simulink model "pathPlanningSimulinkModel"  (R2022b)
settings: Solver=VariableStepAuto  StartTime=0.0  StopTime=inf  RelTol=1e-3
model workspace (MAT data in the model file):
  Sig = Simulink.Signal
  Sig.DataType = 'auto'
  Sig.Dimensions = -1
  Sig.DimensionsMode = 'auto'
  Sig.Complexity = 'auto'
  Sig.SampleTime = -1
  Sig.SamplingMode = 'auto'
values from neighbouring files (symbols this model uses):
  complexMap = [1 1 1 1 1 1 1 1 1 1 1 1 ... (2132 elements, 41x52)]    [matlab.mat]
  r = rateControl(1/sampleTime)    [lidarsensor.m]
undefined symbols (not defined in the file or in its folder): a, b, c, m, n, o, p, q
libraries: robotmobilelib x3, robotalgslib x3
settings Model: Creator=The MathWorks, Inc.  LastModifiedBy=christian.badolo
settings SolverCC: AlgebraicLoopSolver=TrustRegion
settings DebuggingCC: UnconnectedInputMsg=warning  UnconnectedOutputMsg=warning  UnconnectedLineMsg=warning  SymbolicDimsDataTypeCodeGenerationDiagnostic=none  SFMachineParentedDataDiag=warning
settings ModelReferenceCC: EnableRefExpFcnMdlSchedulingChecks=on
settings RTWCC: DLArmComputeVersion=19.05

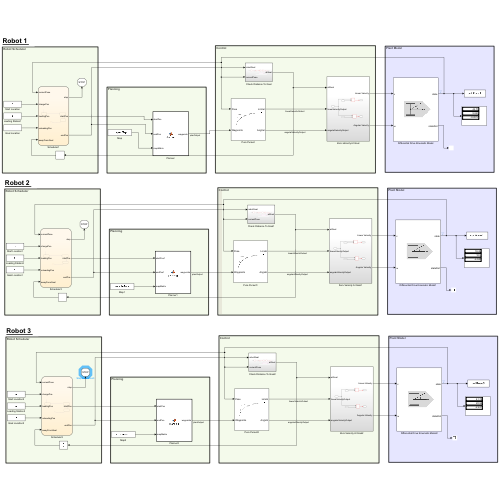
[thumbnail: Simulink's stored preview of the top-level diagram]
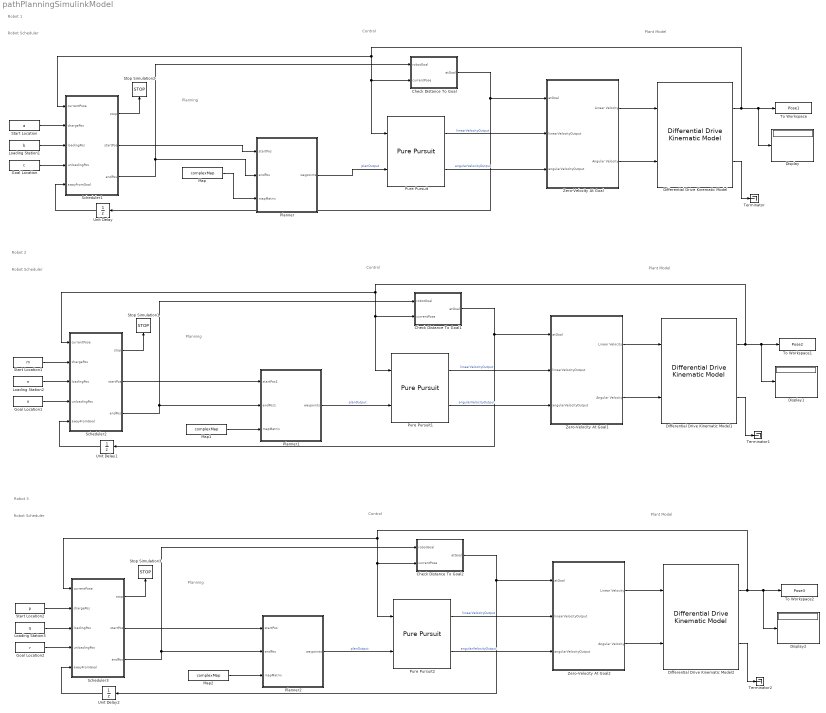
== system pathPlanningSimulinkModel ==
  note: Robot 1
  note: Plant Model
  note: Control
  note: Robot Scheduler
  note: Planning
  note: Plant Model
  note: Planning
  note: Control
  note: Robot Scheduler
  note: Robot 2
  note: Planning
  note: Control
  note: Robot Scheduler
  note: Plant Model
  note: Robot 3
  Check Distance To Goal : Subsystem
  Check Distance To Goal1 : Subsystem
  Check Distance To Goal2 : Subsystem
  Differential Drive Kinematic Model : robotmobilelib/Differential Drive Kinematic Model  VehicleInputs=Vehicle Speed & Heading Angular Velocity  WheelRadius=0.05  WheelSpeedRange=[-inf inf]  TrackWidth=0.2  InitialState=[a, 0]'  SimulateUsing=Interpreted execution
  Differential Drive Kinematic Model1 : robotmobilelib/Differential Drive Kinematic Model  VehicleInputs=Vehicle Speed & Heading Angular Velocity  WheelRadius=0.05  WheelSpeedRange=[-inf inf]  TrackWidth=0.2  InitialState=[m, 0]'  SimulateUsing=Interpreted execution
  Differential Drive Kinematic Model2 : robotmobilelib/Differential Drive Kinematic Model  VehicleInputs=Vehicle Speed & Heading Angular Velocity  WheelRadius=0.05  WheelSpeedRange=[-inf inf]  TrackWidth=0.2  InitialState=[p, 0]'  SimulateUsing=Interpreted execution
  Display : Display
  Display1 : Display
  Display2 : Display
  Goal Location : Constant  Value=c
  Goal Location1 : Constant  Value=o
  Goal Location2 : Constant  Value=r
  Loading Station1 : Constant  Value=b
  Loading Station2 : Constant  Value=n
  Loading Station3 : Constant  Value=q
  Map : Constant  Value=complexMap
  Map1 : Constant  Value=complexMap
  Map2 : Constant  Value=complexMap
  Planner : MATLAB Function  TreatAsAtomicUnit=on
  Planner1 : MATLAB Function  TreatAsAtomicUnit=on
  Planner2 : MATLAB Function  TreatAsAtomicUnit=on
  Pure Pursuit : robotalgslib/Pure Pursuit  DesiredLinearVelocity=0.5  MaxAngularVelocity=1.0  LookaheadDistance=0.5  TargetDirPort=off  SimulateUsing=Code generation
  Pure Pursuit1 : robotalgslib/Pure Pursuit  DesiredLinearVelocity=0.5  MaxAngularVelocity=1.0  LookaheadDistance=0.5  TargetDirPort=off  SimulateUsing=Code generation
  Pure Pursuit2 : robotalgslib/Pure Pursuit  DesiredLinearVelocity=0.2  MaxAngularVelocity=1.0  LookaheadDistance=0.5  TargetDirPort=off  SimulateUsing=Code generation
  Scheduler1 : Stateflow chart  TreatAsAtomicUnit=on
  Scheduler2 : Stateflow chart  TreatAsAtomicUnit=on
  Scheduler3 : Stateflow chart  TreatAsAtomicUnit=on
  Start Location : Constant  Value=a
  Start Location1 : Constant  Value=m
  Start Location2 : Constant  Value=p
  Stop Simulation1 : Stop
  Stop Simulation2 : Stop
  Stop Simulation3 : Stop
  Terminator : Terminator
  Terminator1 : Terminator
  Terminator2 : Terminator
  To Workspace : ToWorkspace  VariableName=Pose1  SampleTime=-1
  To Workspace1 : ToWorkspace  VariableName=Pose2  SampleTime=-1
  To Workspace2 : ToWorkspace  VariableName=Pose3  SampleTime=-1
  Unit Delay : UnitDelay  SampleTime=-1  HasFrameUpgradeWarning=on
  Unit Delay1 : UnitDelay  SampleTime=-1  HasFrameUpgradeWarning=on
  Unit Delay2 : UnitDelay  SampleTime=-1  HasFrameUpgradeWarning=on
  Zero-Velocity At Goal : Subsystem
  Zero-Velocity At Goal1 : Subsystem
  Zero-Velocity At Goal2 : Subsystem
  wires:
  Check Distance To Goal/1(atGoal) -> Unit Delay/1, Zero-Velocity At Goal/1(atGoal)
  Pure Pursuit/1 -> Zero-Velocity At Goal/2(linearVelocityOutput)  "linearVelocityOutput"
  Planner/1(waypoints) -> Pure Pursuit/2  "planOutput"
  Pure Pursuit/2 -> Zero-Velocity At Goal/3(angularVelocityOutput)  "angularVelocityOutput"
  Zero-Velocity At Goal/1(Linear Velocity) -> Differential Drive Kinematic Model/1
  Zero-Velocity At Goal/2(Angular Velocity) -> Differential Drive Kinematic Model/2
  Differential Drive Kinematic Model/2 -> Terminator/1
  Scheduler1/2(startPos) -> Planner/1(startPos)
  Start Location/1 -> Scheduler1/2(chargePos)
  Scheduler1/1(stop) -> Stop Simulation2/1
  Scheduler1/3(endPos) -> Check Distance To Goal/1(robotGoal), Planner/2(endPos)
  Differential Drive Kinematic Model/1 -> To Workspace/1, Display/1, Scheduler1/1(currentPose), Pure Pursuit/1, Check Distance To Goal/2(currentPose)
  Loading Station1/1 -> Scheduler1/3(loadingPos)
  Goal Location/1 -> Scheduler1/4(unloadingPos)
  Unit Delay/1 -> Scheduler1/5(awayFromGoal)
  Map/1 -> Planner/3(mapMatrix)
  Map1/1 -> Planner1/3(mapMatrix)
  Zero-Velocity At Goal1/1(Linear Velocity) -> Differential Drive Kinematic Model1/1
  Loading Station2/1 -> Scheduler2/3(loadingPos)
  Scheduler2/1(stop) -> Stop Simulation1/1
  Scheduler2/3(endPos) -> Planner1/2(endPos1), Check Distance To Goal1/1(robotGoal)
  Planner1/1(waypoints) -> Pure Pursuit1/2  "planOutput"
  Unit Delay1/1 -> Scheduler2/5(awayFromGoal)
  Start Location1/1 -> Scheduler2/2(chargePos)
  Check Distance To Goal1/1(atGoal) -> Unit Delay1/1, Zero-Velocity At Goal1/1(atGoal)
  Zero-Velocity At Goal1/2(Angular Velocity) -> Differential Drive Kinematic Model1/2
  Pure Pursuit1/1 -> Zero-Velocity At Goal1/2(linearVelocityOutput)  "linearVelocityOutput"
  Differential Drive Kinematic Model1/1 -> To Workspace1/1, Display1/1, Scheduler2/1(currentPose), Pure Pursuit1/1, Check Distance To Goal1/2(currentPose)
  Goal Location1/1 -> Scheduler2/4(unloadingPos)
  Differential Drive Kinematic Model1/2 -> Terminator1/1
  Pure Pursuit1/2 -> Zero-Velocity At Goal1/3(angularVelocityOutput)  "angularVelocityOutput"
  Scheduler2/2(startPos) -> Planner1/1(startPos1)
  Planner2/1(waypoints) -> Pure Pursuit2/2  "planOutput"
  Zero-Velocity At Goal2/2(Angular Velocity) -> Differential Drive Kinematic Model2/2
  Scheduler3/1(stop) -> Stop Simulation3/1
  Differential Drive Kinematic Model2/1 -> To Workspace2/1, Display2/1, Scheduler3/1(currentPose), Pure Pursuit2/1, Check Distance To Goal2/2(currentPose)
  Scheduler3/3(endPos) -> Planner2/2(endPos), Check Distance To Goal2/1(robotGoal)
  Pure Pursuit2/1 -> Zero-Velocity At Goal2/2(linearVelocityOutput)  "linearVelocityOutput"
  Scheduler3/2(startPos) -> Planner2/1(startPos)
  Pure Pursuit2/2 -> Zero-Velocity At Goal2/3(angularVelocityOutput)  "angularVelocityOutput"
  Differential Drive Kinematic Model2/2 -> Terminator2/1
  Goal Location2/1 -> Scheduler3/4(unloadingPos)
  Zero-Velocity At Goal2/1(Linear Velocity) -> Differential Drive Kinematic Model2/1
  Check Distance To Goal2/1(atGoal) -> Unit Delay2/1, Zero-Velocity At Goal2/1(atGoal)
  Unit Delay2/1 -> Scheduler3/5(awayFromGoal)
  Loading Station3/1 -> Scheduler3/3(loadingPos)
  Start Location2/1 -> Scheduler3/2(chargePos)
  Map2/1 -> Planner2/3(mapMatrix)

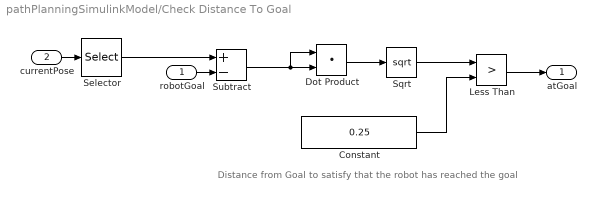
== system pathPlanningSimulinkModel/Check Distance To Goal ==
  note: Distance from Goal to satisfy that the robot has reached the goal
  robotGoal : Inport
  currentPose : Inport  Port=2
  Constant : Constant  Value=0.25
  Dot Product : DotProduct  OutDataTypeStr=Inherit: Inherit via internal rule
  Less Than : RelationalOperator  Operator=>  OutDataTypeStr=boolean  RndMeth=Simplest  InputSameDT=off
  Selector : Selector  InputPortWidth=3  IndexOptions=Index vector (dialog)  Indices=[1 2]  OutputSizes=1
  Sqrt : Sqrt
  Subtract : Sum  Inputs=+-
  atGoal : Outport
  wires:
  robotGoal/1 -> Subtract/2
  Dot Product/1 -> Sqrt/1
  Constant/1 -> Less Than/2
  currentPose/1 -> Selector/1
  Less Than/1 -> atGoal/1
  Sqrt/1 -> Less Than/1
  Subtract/1 -> Dot Product/1, Dot Product/2
  Selector/1 -> Subtract/1

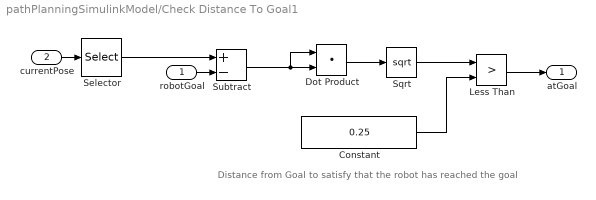
== system pathPlanningSimulinkModel/Check Distance To Goal1 ==
  note: Distance from Goal to satisfy that the robot has reached the goal
  robotGoal : Inport
  currentPose : Inport  Port=2
  Constant : Constant  Value=0.25
  Dot Product : DotProduct  OutDataTypeStr=Inherit: Inherit via internal rule
  Less Than : RelationalOperator  Operator=>  OutDataTypeStr=boolean  RndMeth=Simplest  InputSameDT=off
  Selector : Selector  InputPortWidth=3  IndexOptions=Index vector (dialog)  Indices=[1 2]  OutputSizes=1
  Sqrt : Sqrt
  Subtract : Sum  Inputs=+-
  atGoal : Outport
  wires:
  robotGoal/1 -> Subtract/2
  Dot Product/1 -> Sqrt/1
  Constant/1 -> Less Than/2
  currentPose/1 -> Selector/1
  Less Than/1 -> atGoal/1
  Sqrt/1 -> Less Than/1
  Subtract/1 -> Dot Product/1, Dot Product/2
  Selector/1 -> Subtract/1

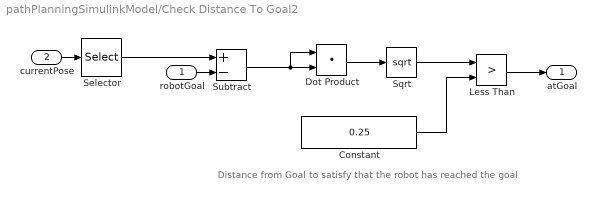
== system pathPlanningSimulinkModel/Check Distance To Goal2 ==
  note: Distance from Goal to satisfy that the robot has reached the goal
  robotGoal : Inport
  currentPose : Inport  Port=2
  Constant : Constant  Value=0.25
  Dot Product : DotProduct  OutDataTypeStr=Inherit: Inherit via internal rule
  Less Than : RelationalOperator  Operator=>  OutDataTypeStr=boolean  RndMeth=Simplest  InputSameDT=off
  Selector : Selector  InputPortWidth=3  IndexOptions=Index vector (dialog)  Indices=[1 2]  OutputSizes=1
  Sqrt : Sqrt
  Subtract : Sum  Inputs=+-
  atGoal : Outport
  wires:
  robotGoal/1 -> Subtract/2
  Dot Product/1 -> Sqrt/1
  Constant/1 -> Less Than/2
  currentPose/1 -> Selector/1
  Less Than/1 -> atGoal/1
  Sqrt/1 -> Less Than/1
  Subtract/1 -> Dot Product/1, Dot Product/2
  Selector/1 -> Subtract/1

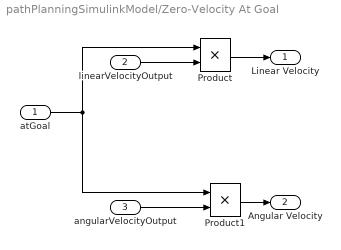
== system pathPlanningSimulinkModel/Zero-Velocity At Goal ==
  atGoal : Inport
  linearVelocityOutput : Inport  Port=2
  angularVelocityOutput : Inport  Port=3
  Product : Product
  Product1 : Product
  Linear Velocity : Outport  OutDataTypeStr=double
  Angular Velocity : Outport  Port=2  OutDataTypeStr=double
  wires:
  atGoal/1 -> Product1/1, Product/1
  angularVelocityOutput/1 -> Product1/2
  linearVelocityOutput/1 -> Product/2
  Product/1 -> Linear Velocity/1
  Product1/1 -> Angular Velocity/1

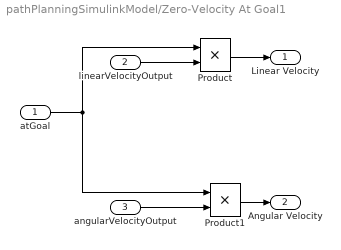
== system pathPlanningSimulinkModel/Zero-Velocity At Goal1 ==
  atGoal : Inport
  linearVelocityOutput : Inport  Port=2
  angularVelocityOutput : Inport  Port=3
  Product : Product
  Product1 : Product
  Linear Velocity : Outport  OutDataTypeStr=double
  Angular Velocity : Outport  Port=2  OutDataTypeStr=double
  wires:
  atGoal/1 -> Product1/1, Product/1
  angularVelocityOutput/1 -> Product1/2
  linearVelocityOutput/1 -> Product/2
  Product/1 -> Linear Velocity/1
  Product1/1 -> Angular Velocity/1

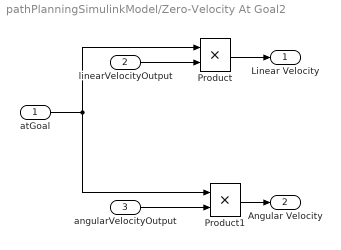
== system pathPlanningSimulinkModel/Zero-Velocity At Goal2 ==
  atGoal : Inport
  linearVelocityOutput : Inport  Port=2
  angularVelocityOutput : Inport  Port=3
  Product : Product
  Product1 : Product
  Linear Velocity : Outport  OutDataTypeStr=double
  Angular Velocity : Outport  Port=2  OutDataTypeStr=double
  wires:
  atGoal/1 -> Product1/1, Product/1
  angularVelocityOutput/1 -> Product1/2
  linearVelocityOutput/1 -> Product/2
  Product/1 -> Linear Velocity/1
  Product1/1 -> Angular Velocity/1

== matlab function pathPlanningSimulinkModel/Planner1 ==
  settings: updateMethod=DISCRETE
  data: startPos1 input size=[1 2]; endPos1 input size=[1 2]; waypoints output size=[2132 2]; mapMatrix input
function waypoints = planning(startPos1, endPos1, mapMatrix)

persistent waypointsInternal
persistent prevStartPos
persistent prevEndPos

% Set constant parameters
maxNumNodes = 2132;

% Initialize persistent variables that are used downstream
if isempty(prevStartPos)
    prevStartPos = startPos1;
end

if isempty(prevEndPos)
    prevEndPos = endPos1;
end

isNewPath = (~isequal(prevStartPos, startPos1) || ~isequal(prevEndPos, endPos1));

if isempty(waypointsInternal) || isNewPath
    % Two conditions in which waypoints must be set: they are not yet
    % initialized, or they are initialized, but the current start and end
    % do not match those used to generate the previous set of waypoints
    [waypointsInternal] = planPath(mapMatrix, maxNumNodes, startPos1, endPos1);
end

% Update the outputs
waypoints = waypointsInternal;

% Update the persistent variables that indicate previous state
prevStartPos = startPos1;
prevEndPos = endPos1;

%% Helper Function

    function wayPoints = planPath(mapMatrix, maxNodes, startPos1, endPos1)
    
    % Create a probabilistic roadmap
    map = binaryOccupancyMap(mapMatrix);
    prm = mobileRobotPRM(map, maxNodes);
    
    % Find a path between two points
    xy = findpath(prm, startPos1, endPos1);
    wayPoints = repmat(endPos1, maxNodes, 1);
    
    % Number of nodes that are actually used
    numNodes = length(xy);
    wayPoints(1:numNodes,:) = xy;    

end

end

== stateflow chart pathPlanningSimulinkModel/Scheduler2 ==
  settings: sampleTime=0.01
  state Unloading
    entry, during:
    endPos = unloadingPos';
  state Loading
    entry,during:
    endPos = loadingPos';
  state Charging
    entry, during:
    endPos = chargePos';
  (default) -> Loading : {startPos = chargePos';}
  Loading -> Unloading : [~awayFromGoal && after(stopDelay, tick)]
      |
      | {startPos = currentPose(1:2)';}
  Unloading -> Charging : [~awayFromGoal  && after(stopDelay, tick)]
      | {startPos = currentPose(1:2)';}
  Charging -> (junction 201) : [~awayFromGoal]{stop = 1;}
  data: currentPose input; stop output =0; chargePos input size=[2 1]; loadingPos input size=[2 1]; unloadingPos input size=[2 1]; startPos output size=[1, 2]; endPos output size=[1, 2]; awayFromGoal input; stopDelay constant double =0.7e2

== matlab function pathPlanningSimulinkModel/Planner ==
  settings: updateMethod=DISCRETE
  data: startPos input size=[1 2]; endPos input size=[1 2]; waypoints output size=[2132 2]; mapMatrix input
function waypoints = planning(startPos, endPos, mapMatrix)

persistent waypointsInternal
persistent prevStartPos
persistent prevEndPos

% Set constant parameters
maxNumNodes = 2132;

% Initialize persistent variables that are used downstream
if isempty(prevStartPos)
    prevStartPos = startPos;
end

if isempty(prevEndPos)
    prevEndPos = endPos;
end

isNewPath = (~isequal(prevStartPos, startPos) || ~isequal(prevEndPos, endPos));

if isempty(waypointsInternal) || isNewPath
    % Two conditions in which waypoints must be set: they are not yet
    % initialized, or they are initialized, but the current start and end
    % do not match those used to generate the previous set of waypoints
    [waypointsInternal] = planPath(mapMatrix, maxNumNodes, startPos, endPos);
end

% Update the outputs
waypoints = waypointsInternal;

% Update the persistent variables that indicate previous state
prevStartPos = startPos;
prevEndPos = endPos;

%% Helper Function

function wayPoints = planPath(mapMatrix, maxNodes, startPos, endPos)
    
    % Create a probabilistic roadmap
    map = binaryOccupancyMap(mapMatrix);
    prm = mobileRobotPRM(map, maxNodes);
    
    % Find a path between two points
    xy = findpath(prm, startPos, endPos);
    wayPoints = repmat(endPos, maxNodes, 1);
    
    % Number of nodes that are actually used
    numNodes = length(xy);
    wayPoints(1:numNodes,:) = xy;    

end

end

== stateflow chart pathPlanningSimulinkModel/Scheduler1 ==
  settings: sampleTime=0.01
  state Unloading
    entry, during:
    endPos = unloadingPos';
  state Loading
    entry,during:
    endPos = loadingPos';
  state Charging
    entry, during:
    endPos = chargePos';
  (default) -> Loading : {startPos = chargePos';}
  Loading -> Unloading : [~awayFromGoal && after(stopDelay, tick)]
      |
      | {startPos = currentPose(1:2)';}
  Unloading -> Charging : [~awayFromGoal  && after(stopDelay, tick)]
      | {startPos = currentPose(1:2)';}
  Charging -> (junction 201) : [~awayFromGoal]{stop = 1;}
  data: currentPose input; stop output =0; chargePos input size=[2 1]; loadingPos input size=[2 1]; unloadingPos input size=[2 1]; startPos output size=[1, 2]; endPos output size=[1, 2]; awayFromGoal input; stopDelay constant double =0.7e1

== matlab function pathPlanningSimulinkModel/Planner2 ==
  settings: updateMethod=DISCRETE
  data: startPos input size=[1 2]; endPos input size=[1 2]; waypoints output size=[2132 2]; mapMatrix input
function waypoints = planning(startPos, endPos, mapMatrix)

persistent waypointsInternal
persistent prevStartPos
persistent prevEndPos

% Set constant parameters
maxNumNodes = 2132;

% Initialize persistent variables that are used downstream
if isempty(prevStartPos)
    prevStartPos = startPos;
end

if isempty(prevEndPos)
    prevEndPos = endPos;
end

isNewPath = (~isequal(prevStartPos, startPos) || ~isequal(prevEndPos, endPos));

if isempty(waypointsInternal) || isNewPath
    % Two conditions in which waypoints must be set: they are not yet
    % initialized, or they are initialized, but the current start and end
    % do not match those used to generate the previous set of waypoints
    [waypointsInternal] = planPath(mapMatrix, maxNumNodes, startPos, endPos);
end

% Update the outputs
waypoints = waypointsInternal;

% Update the persistent variables that indicate previous state
prevStartPos = startPos;
prevEndPos = endPos;

%% Helper Function

function wayPoints = planPath(mapMatrix, maxNodes, startPos, endPos)
    
    % Create a probabilistic roadmap
    map = binaryOccupancyMap(mapMatrix);
    prm = mobileRobotPRM(map, maxNodes);
    
    % Find a path between two points
    xy = findpath(prm, startPos, endPos);
    wayPoints = repmat(endPos, maxNodes, 1);
    
    % Number of nodes that are actually used
    numNodes = length(xy);
    wayPoints(1:numNodes,:) = xy;    

end

end

== stateflow chart pathPlanningSimulinkModel/Scheduler3 ==
  settings: sampleTime=0.01
  state Unloading
    entry, during:
    endPos = unloadingPos';
  state Loading
    entry,during:
    endPos = loadingPos';
  state Charging
    entry, during:
    endPos = chargePos';
  (default) -> Loading : {startPos = chargePos';}
  Loading -> Unloading : [~awayFromGoal && after(stopDelay, tick)]
      |
      | {startPos = currentPose(1:2)';}
  Unloading -> Charging : [~awayFromGoal  && after(stopDelay, tick)]
      | {startPos = currentPose(1:2)';}
  Charging -> (junction 201) : [~awayFromGoal]{stop = 1;}
  data: currentPose input; stop output =0; chargePos input size=[2 1]; loadingPos input size=[2 1]; unloadingPos input size=[2 1]; startPos output size=[1, 2]; endPos output size=[1, 2]; awayFromGoal input; stopDelay constant double =0.7e2
